simulink model "MassDamperSystem"  (R2020a)
settings: Solver=FixedStepAuto  StartTime=0.0  StopTime=10.0  FixedStep=0.1  RelTol=1e-3
model workspace (MAT data in the model file):
  c = Simulink.Parameter
  c.Value = 3
  c.Description = 'Damping coefficient'
  c.DataType = 'double'
  c.DocUnits = 'Ns/m'
  c.Dimensions = [1 1]
  k = Simulink.Parameter
  k.Value = 50
  k.DataType = 'auto'
  k.DocUnits = 'N/m'
  k.Dimensions = [1 1]
  m = Simulink.Parameter
  m.Value = 5
  m.DataType = 'auto'
  m.DocUnits = 'kg'
  m.Dimensions = [1 1]
  v0 = Simulink.Parameter
  v0.Value = 10
  v0.DataType = 'auto'
  v0.DocUnits = 'm/s'
  v0.Dimensions = [1 1]
settings Model: SnapshotInterval=1  EnablePacing=on  OrderedModelArguments=off  Creator=13ann  LastModifiedBy=13ann

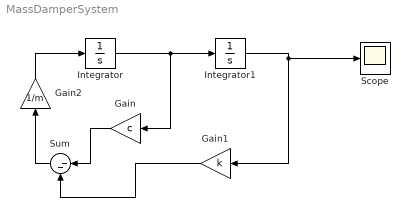
== system MassDamperSystem ==
  Gain : Gain  Gain=c
  Gain1 : Gain  Gain=k
  Gain2 : Gain  Gain=1/m
  Integrator : Integrator  InitialCondition=v0
  Integrator1 : Integrator
  Scope : Scope
  Sum : Sum  Inputs=|--
  wires:
  Integrator/1 -> Gain/1, Integrator1/1
  Integrator1/1 -> Scope/1, Gain1/1
  Sum/1 -> Gain2/1
  Gain2/1 -> Integrator/1
  Gain1/1 -> Sum/2
  Gain/1 -> Sum/1
